simulink model "simulation_system"  (R2015a)
settings: Solver=ode45  StartTime=0.0  StopTime=10  RelTol=1e-3
values from neighbouring files (symbols this model uses):
  Ad = Gd.den{:}    [modelisation_MCC.m]
  Bd = Gd.num{:}    [modelisation_MCC.m]
  Fd = c2d(Fc,Te)    [modelisation_MCC.m]
  Kf = 1/dcgain(Fd)    [modelisation_MCC.m]
  Rd = conv(S,Dr)    [modelisation_MCC.m]
  Rn = (conv(R,Dc))'    [modelisation_MCC.m]
  T = (1/sum(Bd))*P    [modelisation_MCC.m]
  Te = 0.02    [Courbe_test.m]    (also in modelisation_MCC.m = 0.03)
settings Model: CovSFcnEnable=off  Creator=diallocherif  LastModifiedBy=mbemb_000
settings DebuggingCC: SolverPrmCheckMsg=warning

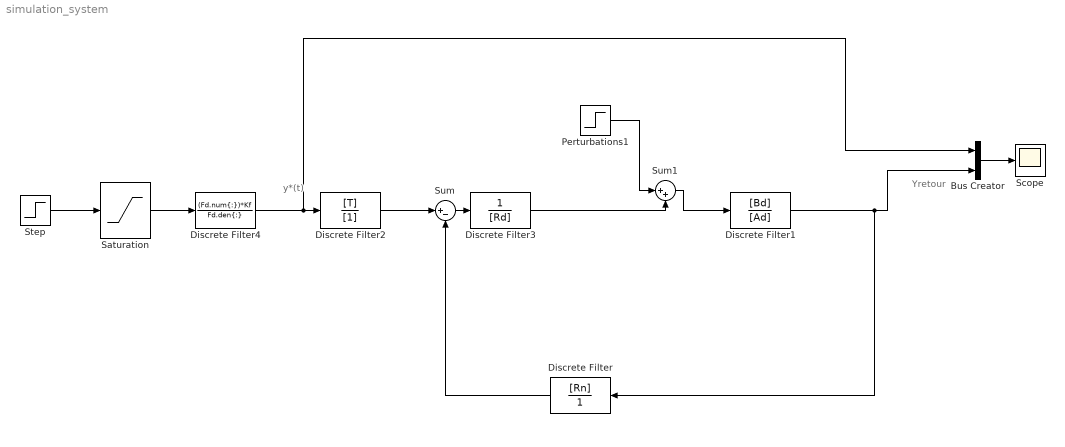
== system simulation_system ==
  note: Yretour
  note: y*(t)
  Bus Creator : BusCreator  Inputs=2
  Discrete Filter : DiscreteFilter  Numerator=[Rn]  Denominator=1  SampleTime=Te
  Discrete Filter1 : DiscreteFilter  Numerator=[Bd]  Denominator=[Ad]  SampleTime=Te
  Discrete Filter2 : DiscreteFilter  Numerator=[T]  Denominator=[1]  SampleTime=Te
  Discrete Filter3 : DiscreteFilter  Numerator=1  Denominator=[Rd]  SampleTime=Te
  Discrete Filter4 : DiscreteFilter  Numerator=(Fd.num{:})*Kf  Denominator=Fd.den{:}  SampleTime=Te
  Perturbations1 : Step  Time=3  SampleTime=Te
  Saturation : Saturate  UpperLimit=1  LowerLimit=-1
  Scope : Scope
      settings: YMin=-1  YMax=1
  Step : Step  After=2  SampleTime=Te
  Sum : Sum  Inputs=|+-
  Sum1 : Sum  Inputs=|++
  wires:
  Discrete Filter2/1 -> Sum/1
  Discrete Filter/1 -> Sum/2
  Sum/1 -> Discrete Filter3/1
  Bus Creator/1 -> Scope/1
  Discrete Filter4/1 -> Bus Creator/1, Discrete Filter2/1
  Step/1 -> Saturation/1
  Sum1/1 -> Discrete Filter1/1
  Discrete Filter3/1 -> Sum1/2
  Saturation/1 -> Discrete Filter4/1
  Discrete Filter1/1 -> Discrete Filter/1, Bus Creator/2
  Perturbations1/1 -> Sum1/1
